simulink model "HopfMapEquationTB"  (R2020a)
settings: Solver=VariableStepAuto  StartTime=0.0  StopTime=10.0  RelTol=1e-3
undefined symbols (not defined in the file): magnitude
settings Model: Creator=finla  LastModifiedBy=finla

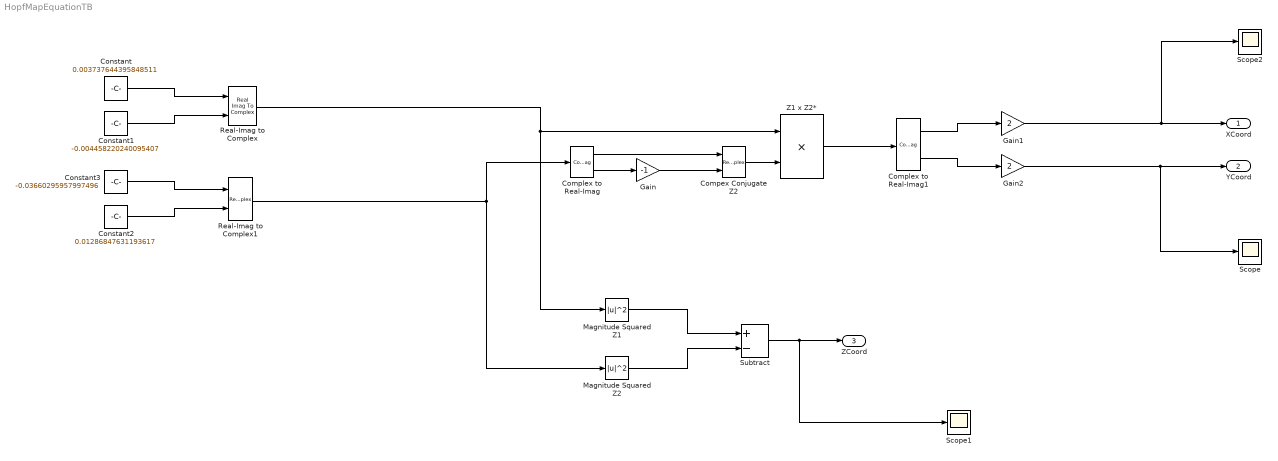
== system HopfMapEquationTB ==
  Compex Conjugate Z2 : RealImagToComplex
  Complex to Real-Imag : ComplexToRealImag
  Complex to Real-Imag1 : ComplexToRealImag
  Constant : Constant  Value=0.003737644395848511  OutDataTypeStr=fixdt(1,22,20)
  Constant1 : Constant  Value=-0.004458220240095407  OutDataTypeStr=fixdt(1,22,20)
  Constant2 : Constant  Value=0.01286847631193617  OutDataTypeStr=fixdt(1,22,20)
  Constant3 : Constant  Value=-0.03660295957997496  OutDataTypeStr=fixdt(1,22,20)
  Gain : Gain  Gain=-1  OutDataTypeStr=fixdt(1,22,20)  SaturateOnIntegerOverflow=on
  Gain1 : Gain  Gain=2  OutDataTypeStr=fixdt(1,22,20)  SaturateOnIntegerOverflow=on
  Gain2 : Gain  Gain=2  OutDataTypeStr=fixdt(1,22,20)  SaturateOnIntegerOverflow=on
  Magnitude Squared Z1 : Math  Operator=magnitude^2  OutDataTypeStr=fixdt(1,22,20)  SaturateOnIntegerOverflow=on
  Magnitude Squared Z2 : Math  Operator=magnitude^2  OutDataTypeStr=fixdt(1,22,20)  SaturateOnIntegerOverflow=on
  Real-Imag to Complex : RealImagToComplex
  Real-Imag to Complex1 : RealImagToComplex
  Scope : Scope
  Scope1 : Scope
  Scope2 : Scope
  Subtract : Sum  Inputs=+-  AccumDataTypeStr=fixdt(1,32,20)
  Z1 x Z2* : Product  OutDataTypeStr=fixdt(1,22,20)
  XCoord : Outport  OutDataTypeStr=fixdt(1,22,20)
  YCoord : Outport  Port=2  OutDataTypeStr=fixdt(1,22,20)
  ZCoord : Outport  Port=3  OutDataTypeStr=fixdt(1,32,20)
  wires:
  Complex to Real-Imag1/2 -> Gain2/1
  Gain1/1 -> Scope2/1, XCoord/1
  Gain2/1 -> Scope/1, YCoord/1
  Z1 x Z2*/1 -> Complex to Real-Imag1/1
  Complex to Real-Imag/2 -> Gain/1
  Magnitude Squared Z1/1 -> Subtract/1
  Real-Imag to Complex1/1 -> Complex to Real-Imag/1, Magnitude Squared Z2/1
  Real-Imag to Complex/1 -> Magnitude Squared Z1/1, Z1 x Z2*/1
  Magnitude Squared Z2/1 -> Subtract/2
  Gain/1 -> Compex Conjugate Z2/2
  Complex to Real-Imag1/1 -> Gain1/1
  Complex to Real-Imag/1 -> Compex Conjugate Z2/1
  Subtract/1 -> Scope1/1, ZCoord/1
  Compex Conjugate Z2/1 -> Z1 x Z2*/2
  Constant3/1 -> Real-Imag to Complex1/1
  Constant2/1 -> Real-Imag to Complex1/2
  Constant/1 -> Real-Imag to Complex/1
  Constant1/1 -> Real-Imag to Complex/2
